simulink model "MotorControl"  (R2023b)
settings: Solver=FixedStepDiscrete  StartTime=0.0  StopTime=8  FixedStep=1e-5  RelTol=1e-3
libraries: slpidlib x2, autolibpmsminterior x1, autolibinverter x1
settings Model: Creator=Elio  LastModifiedBy=Elio

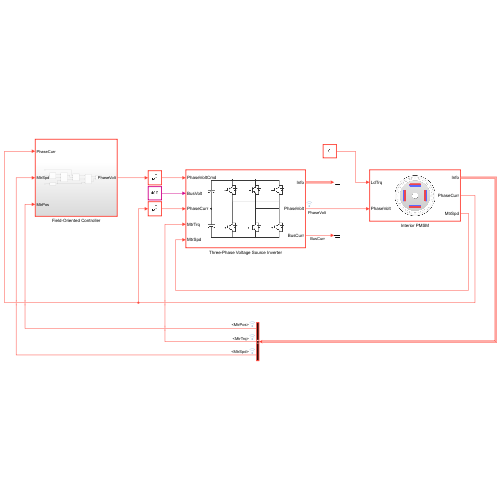
[thumbnail: Simulink's stored preview of the top-level diagram]
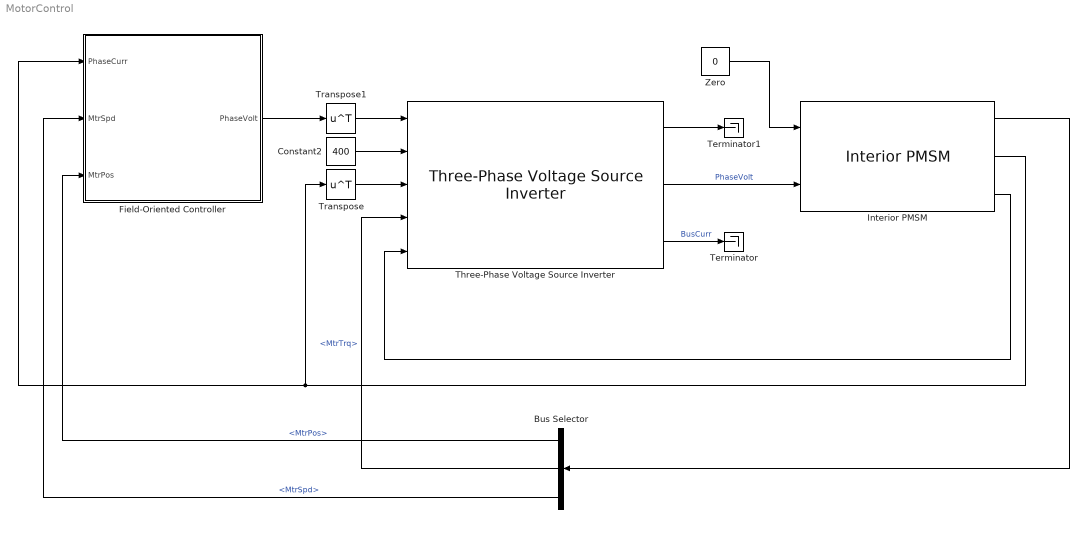
== system MotorControl ==
  Bus Selector : BusSelector  OutputSignals=MtrPos,MtrTrq,MtrSpd
  Constant2 : Constant  Value=400
  Field-Oriented Controller : Subsystem
  Interior PMSM : autolibpmsminterior/Interior PMSM  port_config=Torque  sim_type=Discrete  Ts=1e-5  FilePath=interiorpmsm_motordata.m  P=6  Rs=0.00423  Ldq=[0.171e-3 0.391e-3]  KConstText=Back-emf constant (Ke):  lambda_pm=0.1194  Ke=59.16664  mechanical=[0.0036, 0.0011, 0]  idq0=[0 0]  theta_init=0  omega_init=0  KConst=59.16664  lambda_pm_calc=0.054367  Kt=1.323  RefBlkName='autolibpmsminterior/Interior PMSM'  aMode=1
      settings: LibrarySourceBlock=autolibemachines/Interior PMSM
  Terminator : Terminator
  Terminator1 : Terminator
  Three-Phase Voltage Source Inverter : autolibinverter/Three-Phase Voltage Source Inverter  InvrtrTmpInpEnbl=off  enable_hdl=off  model_type=Commanded phase voltage  fs=10000  w_eff_bp=[-1000 -500 0 500 1000]  n1=128  T_eff_bp=[-200 -100 0 100 200]  Temp_eff_bp=[213.15 293.15 373.15]  n2=128  ploss_table=[1 0.999 0.989 0.997 0.996;0.995 0.994 0.993 0.992 0.991;0.990 0.989 0.988 0.987 0.986;0.985 0.984 0.983 0.982 0.981;0.980 0.979 0.978 0.977 0.976]  ploss_table_3d=cat(3,0.95*[1 0.999 0.989 0.997 0.996;0.995 0.994 0.993 0.992 0.991;0.990 0.989 0.988 0.987 0.986;0.985 0.984 0.983 0.982 0.981;0.980 0.979 0.978 0.977 0.976],[1 0.999 0.989 0.997 0.996;0.995 0.994 0.993 0.992 0.991;0.990 0.989 0.988 0.987 0.986;0.985 0.984 0.983 0.982 0.981;0.980 0.979 0.978 0.977 0.976],0.92*[1 0.999 0.989 0.997 0.996;0.995 0.994 0.993 0.992 0.991;0.990 0.989 0.988 0.987 0.986;0.985 0.984 0.983 0.982 0.981;0.980 0.979 0.978 0.977 0.976])  preExtrapFlag=off  u1max=1000  u1min=-1000  u2max=200  u2min=-200  intPrec=23  RefBlkName='autolibmappedmotor/Mapped Motor'  CalLossMapData={}  CalLossWithTempMapData={}
      settings: LibrarySourceBlock=autolibemachines/Three-Phase Voltage Source Inverter
  Transpose : Math  Operator=transpose
  Transpose1 : Math  Operator=transpose
  Zero : Constant  Value=0  OutDataTypeStr=Inherit: Inherit via back propagation  SampleTime=1e-5
  wires:
  Zero/1 -> Interior PMSM/1
  Interior PMSM/2 -> Transpose/1, Field-Oriented Controller/1(PhaseCurr)
  Three-Phase Voltage Source Inverter/2 -> Interior PMSM/2  "PhaseVolt"
  Bus Selector/1 -> Field-Oriented Controller/3(MtrPos)  "<MtrPos>"
  Three-Phase Voltage Source Inverter/1 -> Terminator1/1
  Bus Selector/3 -> Field-Oriented Controller/2(MtrSpd)  "<MtrSpd>"
  Transpose/1 -> Three-Phase Voltage Source Inverter/3
  Bus Selector/2 -> Three-Phase Voltage Source Inverter/4  "<MtrTrq>"
  Transpose1/1 -> Three-Phase Voltage Source Inverter/1
  Constant2/1 -> Three-Phase Voltage Source Inverter/2
  Three-Phase Voltage Source Inverter/3 -> Terminator/1  "BusCurr"
  Field-Oriented Controller/1(PhaseVolt) -> Transpose1/1
  Interior PMSM/3 -> Three-Phase Voltage Source Inverter/5
  Interior PMSM/1 -> Bus Selector/1

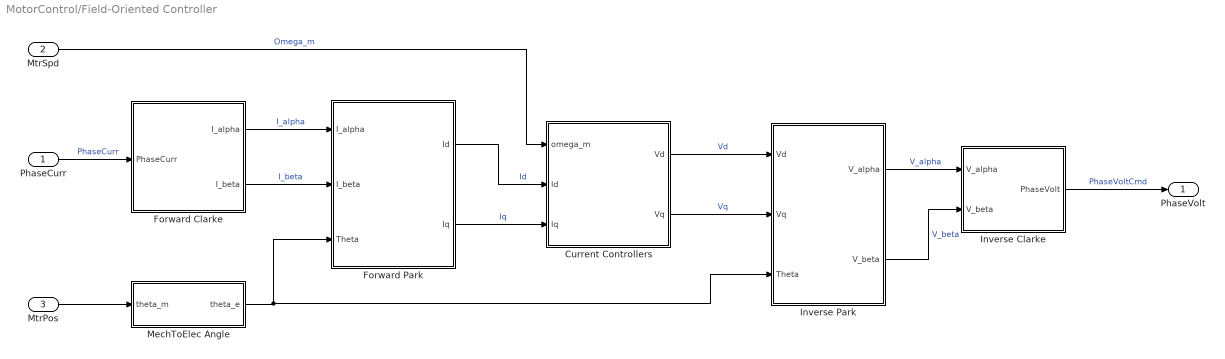
== system MotorControl/Field-Oriented Controller ==
  PhaseCurr : Inport
  MtrSpd : Inport  Port=2
  MtrPos : Inport  Port=3
  Current Controllers : Subsystem
  Forward Clarke : Subsystem
  Forward Park : Subsystem
  Inverse Clarke : Subsystem
  Inverse Park : Subsystem
  MechToElec Angle : Subsystem
  PhaseVolt : Outport
  wires:
  PhaseCurr/1 -> Forward Clarke/1(PhaseCurr)  "PhaseCurr"
  Forward Clarke/1(I_alpha) -> Forward Park/1(I_alpha)  "I_alpha"
  Forward Clarke/2(I_beta) -> Forward Park/2(I_beta)  "I_beta"
  MtrPos/1 -> MechToElec Angle/1(theta_m)
  Inverse Clarke/1(PhaseVolt) -> PhaseVolt/1  "PhaseVoltCmd"
  MtrSpd/1 -> Current Controllers/1(omega_m)  "Omega_m"
  Inverse Park/2(V_beta) -> Inverse Clarke/2(V_beta)  "V_beta"
  Inverse Park/1(V_alpha) -> Inverse Clarke/1(V_alpha)  "V_alpha"
  Forward Park/1(Id) -> Current Controllers/2(Id)  "Id"
  Forward Park/2(Iq) -> Current Controllers/3(Iq)  "Iq"
  Current Controllers/1(Vd) -> Inverse Park/1(Vd)  "Vd"
  Current Controllers/2(Vq) -> Inverse Park/2(Vq)  "Vq"
  MechToElec Angle/1(theta_e) -> Forward Park/3(Theta), Inverse Park/3(Theta)

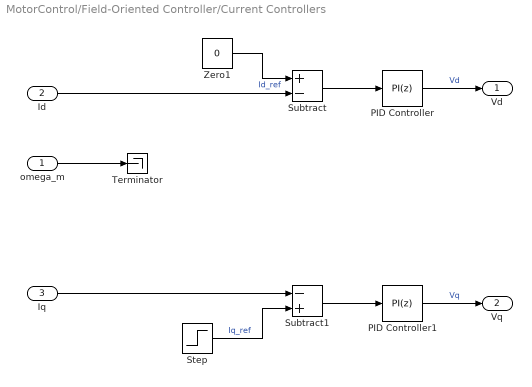
== system MotorControl/Field-Oriented Controller/Current Controllers ==
  omega_m : Inport
  Id : Inport  Port=2
  Iq : Inport  Port=3
  PID Controller : slpidlib/PID Controller  Controller=PI  Form=Parallel  TimeDomain=Discrete-time  UseExternalTs=off  SampleTime=1e-5  IntegratorMethod=Forward Euler  FilterMethod=Forward Euler  ControllerParametersSource=internal  P=13.4666695236978  I=8567.48164264561  UseKiTs=off  D=0  N=100  UseFilter=on  TunerSelectOption=Transfer Function Based (PID Tuner App)  InitialConditionSource=internal  InitialConditionForIntegrator=0  InitialConditionForFilter=0  DifferentiatorICPrevScaledInput=0  ExternalReset=none  TrackingMode=off  Kt=1  LimitOutput=off  SatLimitsSource=internal  UpperSaturationLimit=inf  LowerSaturationLimit=-inf  LinearizeAsGain=on  AntiWindupMode=none  Kb=1  LimitIntegrator=off  UpperIntegratorSaturationLimit=inf  LowerIntegratorSaturationLimit=-inf  POutMin=[]  POutMax=[]  IOutMin=[]  IOutMax=[]  DOutMin=[]  DOutMax=[]  NOutMin=[]  NOutMax=[]  SumOutMin=[]  SumOutMax=[]  SaturationOutMin=[]  SaturationOutMax=[]  PParamMin=[]  PParamMax=[]  IParamMin=[]  IParamMax=[]  DParamMin=[]  DParamMax=[]  NParamMin=[]  NParamMax=[]  KbParamMin=[]  KbParamMax=[]  KtParamMin=[]  KtParamMax=[]  KbOutMin=[]  KbOutMax=[]  KtOutMin=[]  KtOutMax=[]  IntegratorOutMin=[]  IntegratorOutMax=[]  FilterOutMin=[]  FilterOutMax=[]  SumI1OutMin=[]  SumI1OutMax=[]  SumI2OutMin=[]  SumI2OutMax=[]  SumI3OutMin=[]  SumI3OutMax=[]  SumI4OutMin=[]  SumI4OutMax=[]  SumDOutMin=[]  SumDOutMax=[]  DifferentiatorOutMin=[]  DifferentiatorOutMax=[]  FilterDiffOutCoefMin=[]  FilterDiffOutCoefMax=[]  ReciprocalOutMin=[]  ReciprocalOutMax=[]  SumDenOutMin=[]  SumDenOutMax=[]  SumNumOutMin=[]  SumNumOutMax=[]  DivideOutMin=[]  DivideOutMax=[]  UdiffTsProdOutMin=[]  UdiffTsProdOutMax=[]  NTsProdOutMin=[]  NTsProdOutMax=[]  UintegralTsProdOutMin=[]  UintegralTsProdOutMax=[]  UngainTsProdOutMin=[]  UngainTsProdOutMax=[]  ClampingZeroOutDataTypeStr=Inherit: Inherit via back propagation  ClampingZeroOutMin=[]  ClampingZeroOutMax=[]  FilterDenConstantOutDataTypeStr=Inherit: Inherit via back propagation  FilterDenConstantOutMin=[]  FilterDenConstantOutMax=[]  PCopyOutDataTypeStr=Inherit: Inherit via back propagation  PCopyOutMin=[]  PCopyOutMax=[]  NCopyOutDataTypeStr=Inherit: Inherit via back propagation  NCopyOutMin=[]  NCopyOutMax=[]  IntegratorContinuousStateAttributes=''  IntegratorStateMustResolveToSignalObject=off  IntegratorRTWStateStorageClass=Auto  FilterContinuousStateAttributes=''  FilterStateMustResolveToSignalObject=off  FilterRTWStateStorageClass=Auto  ParallelPVariant=InternalParameters  IdealPVariant=Disabled  IVariant=InternalParameters  DVariant=Disabled  IntegratorVariant=Discrete  SatVariant=Disabled  AWVariant=Passthrough  PCopyVariant=Disabled  TRVariant=Disabled  FdbkBlocksVariant=Forward  IdealPFdbkVariant=Disabled  SatFdbkVariant=Disabled  DerivativeFilterVariant=Disabled  NVariant=Disabled  NCopyVariant=Disabled_SignalSpec  FilterICVariant=Disabled  IntegratorICVariant=InternalICs  ExternalResetVariant=Disabled  TRSumVariant=Passthrough  SumFdbkVariant=Disabled  SumVariant=Sum_PI  TsampFilterVariant=InternalTs  TsampNgainVariant=Passthrough  TsampIntegralVariant=Disabled_SignalSpec  ExternalSaturationOutDataTypeStr=Inherit: Same as second input
  PID Controller1 : slpidlib/PID Controller  Controller=PI  Form=Parallel  TimeDomain=Discrete-time  UseExternalTs=off  SampleTime=1e-5  IntegratorMethod=Forward Euler  FilterMethod=Forward Euler  ControllerParametersSource=internal  P=25  I=13000  UseKiTs=off  D=0  N=100  UseFilter=on  TunerSelectOption=Transfer Function Based (PID Tuner App)  InitialConditionSource=internal  InitialConditionForIntegrator=0  InitialConditionForFilter=0  DifferentiatorICPrevScaledInput=0  ExternalReset=none  TrackingMode=off  Kt=1  LimitOutput=off  SatLimitsSource=internal  UpperSaturationLimit=inf  LowerSaturationLimit=-inf  LinearizeAsGain=on  AntiWindupMode=none  Kb=1  LimitIntegrator=off  UpperIntegratorSaturationLimit=inf  LowerIntegratorSaturationLimit=-inf  POutMin=[]  POutMax=[]  IOutMin=[]  IOutMax=[]  DOutMin=[]  DOutMax=[]  NOutMin=[]  NOutMax=[]  SumOutMin=[]  SumOutMax=[]  SaturationOutMin=[]  SaturationOutMax=[]  PParamMin=[]  PParamMax=[]  IParamMin=[]  IParamMax=[]  DParamMin=[]  DParamMax=[]  NParamMin=[]  NParamMax=[]  KbParamMin=[]  KbParamMax=[]  KtParamMin=[]  KtParamMax=[]  KbOutMin=[]  KbOutMax=[]  KtOutMin=[]  KtOutMax=[]  IntegratorOutMin=[]  IntegratorOutMax=[]  FilterOutMin=[]  FilterOutMax=[]  SumI1OutMin=[]  SumI1OutMax=[]  SumI2OutMin=[]  SumI2OutMax=[]  SumI3OutMin=[]  SumI3OutMax=[]  SumI4OutMin=[]  SumI4OutMax=[]  SumDOutMin=[]  SumDOutMax=[]  DifferentiatorOutMin=[]  DifferentiatorOutMax=[]  FilterDiffOutCoefMin=[]  FilterDiffOutCoefMax=[]  ReciprocalOutMin=[]  ReciprocalOutMax=[]  SumDenOutMin=[]  SumDenOutMax=[]  SumNumOutMin=[]  SumNumOutMax=[]  DivideOutMin=[]  DivideOutMax=[]  UdiffTsProdOutMin=[]  UdiffTsProdOutMax=[]  NTsProdOutMin=[]  NTsProdOutMax=[]  UintegralTsProdOutMin=[]  UintegralTsProdOutMax=[]  UngainTsProdOutMin=[]  UngainTsProdOutMax=[]  ClampingZeroOutDataTypeStr=Inherit: Inherit via back propagation  ClampingZeroOutMin=[]  ClampingZeroOutMax=[]  FilterDenConstantOutDataTypeStr=Inherit: Inherit via back propagation  FilterDenConstantOutMin=[]  FilterDenConstantOutMax=[]  PCopyOutDataTypeStr=Inherit: Inherit via back propagation  PCopyOutMin=[]  PCopyOutMax=[]  NCopyOutDataTypeStr=Inherit: Inherit via back propagation  NCopyOutMin=[]  NCopyOutMax=[]  IntegratorContinuousStateAttributes=''  IntegratorStateMustResolveToSignalObject=off  IntegratorRTWStateStorageClass=Auto  FilterContinuousStateAttributes=''  FilterStateMustResolveToSignalObject=off  FilterRTWStateStorageClass=Auto  ParallelPVariant=InternalParameters  IdealPVariant=Disabled  IVariant=InternalParameters  DVariant=Disabled  IntegratorVariant=Discrete  SatVariant=Disabled  AWVariant=Passthrough  PCopyVariant=Disabled  TRVariant=Disabled  FdbkBlocksVariant=Forward  IdealPFdbkVariant=Disabled  SatFdbkVariant=Disabled  DerivativeFilterVariant=Disabled  NVariant=Disabled  NCopyVariant=Disabled_SignalSpec  FilterICVariant=Disabled  IntegratorICVariant=InternalICs  ExternalResetVariant=Disabled  TRSumVariant=Passthrough  SumFdbkVariant=Disabled  SumVariant=Sum_PI  TsampFilterVariant=InternalTs  TsampNgainVariant=Passthrough  TsampIntegralVariant=Disabled_SignalSpec  ExternalSaturationOutDataTypeStr=Inherit: Same as second input
  Step : Step  After=30  SampleTime=1e-5
  Subtract : Sum  Inputs=+-
  Subtract1 : Sum  Inputs=-+
  Terminator : Terminator
  Zero1 : Constant  Value=0  OutDataTypeStr=Inherit: Inherit via back propagation
  Vd : Outport
  Vq : Outport  Port=2
  wires:
  Subtract1/1 -> PID Controller1/1
  Step/1 -> Subtract1/2  "Iq_ref"
  Zero1/1 -> Subtract/1  "Id_ref"
  Subtract/1 -> PID Controller/1
  Id/1 -> Subtract/2
  Iq/1 -> Subtract1/1
  PID Controller/1 -> Vd/1  "Vd"
  PID Controller1/1 -> Vq/1  "Vq"
  omega_m/1 -> Terminator/1

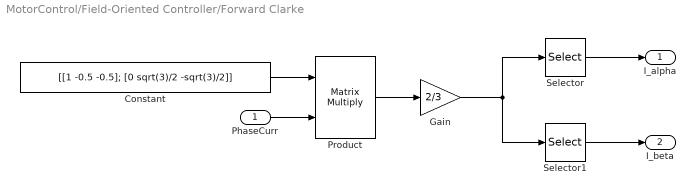
== system MotorControl/Field-Oriented Controller/Forward Clarke ==
  PhaseCurr : Inport
  Constant : Constant  Value=[[1 -0.5 -0.5]; [0 sqrt(3)/2 -sqrt(3)/2]]  SampleTime=1e-5
  Gain : Gain  Gain=2/3
  Product : Product  Multiplication=Matrix(*)
  Selector : Selector  InputPortWidth=2  IndexOptions=Index vector (dialog)  Indices=1  OutputSizes=1
  Selector1 : Selector  InputPortWidth=2  IndexOptions=Index vector (dialog)  Indices=2  OutputSizes=1
  I_alpha : Outport
  I_beta : Outport  Port=2
  wires:
  Constant/1 -> Product/1
  Product/1 -> Gain/1
  Gain/1 -> Selector1/1, Selector/1
  Selector/1 -> I_alpha/1
  Selector1/1 -> I_beta/1
  PhaseCurr/1 -> Product/2

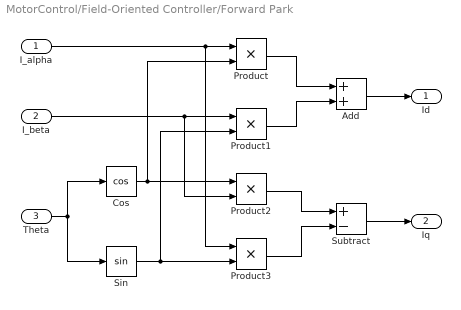
== system MotorControl/Field-Oriented Controller/Forward Park ==
  I_alpha : Inport
  I_beta : Inport  Port=2
  Theta : Inport  Port=3
  Add : Sum
  Cos : Trigonometry  Operator=cos
  Product{,1..3} (4 alike) : Product
  Sin : Trigonometry
  Subtract : Sum  Inputs=+-
  Id : Outport
  Iq : Outport  Port=2
  wires:
  Theta/1 -> Sin/1, Cos/1
  I_alpha/1 -> Product/1, Product3/1
  Cos/1 -> Product2/1, Product/2
  I_beta/1 -> Product1/1, Product2/2
  Sin/1 -> Product3/2, Product1/2
  Product/1 -> Add/1
  Product1/1 -> Add/2
  Add/1 -> Id/1
  Product2/1 -> Subtract/1
  Product3/1 -> Subtract/2
  Subtract/1 -> Iq/1

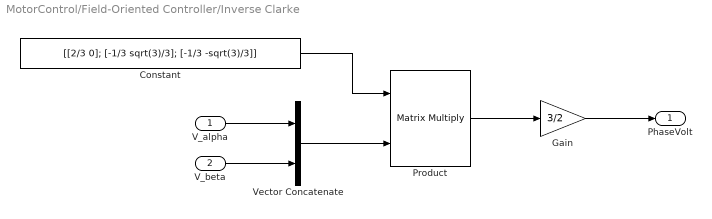
== system MotorControl/Field-Oriented Controller/Inverse Clarke ==
  V_alpha : Inport
  V_beta : Inport  Port=2
  Constant : Constant  Value=[[2/3 0]; [-1/3 sqrt(3)/3]; [-1/3 -sqrt(3)/3]]  SampleTime=1e-5
  Gain : Gain  Gain=3/2
  Product : Product  Multiplication=Matrix(*)
  Vector Concatenate : Concatenate
  PhaseVolt : Outport
  wires:
  V_alpha/1 -> Vector Concatenate/1
  V_beta/1 -> Vector Concatenate/2
  Vector Concatenate/1 -> Product/2
  Constant/1 -> Product/1
  Product/1 -> Gain/1
  Gain/1 -> PhaseVolt/1

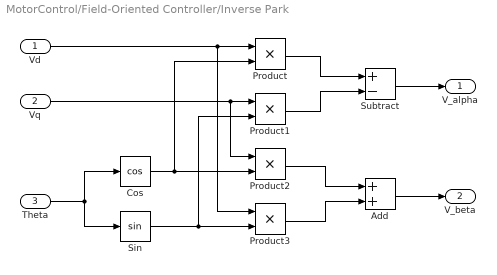
== system MotorControl/Field-Oriented Controller/Inverse Park ==
  Vd : Inport
  Vq : Inport  Port=2
  Theta : Inport  Port=3
  Add : Sum
  Cos : Trigonometry  Operator=cos
  Product{,1..3} (4 alike) : Product
  Sin : Trigonometry
  Subtract : Sum  Inputs=+-
  V_alpha : Outport
  V_beta : Outport  Port=2
  wires:
  Theta/1 -> Cos/1, Sin/1
  Vd/1 -> Product3/1, Product/1
  Cos/1 -> Product/2, Product2/2
  Vq/1 -> Product2/1, Product1/1
  Sin/1 -> Product1/2, Product3/2
  Product/1 -> Subtract/1
  Product1/1 -> Subtract/2
  Subtract/1 -> V_alpha/1
  Product2/1 -> Add/1
  Product3/1 -> Add/2
  Add/1 -> V_beta/1

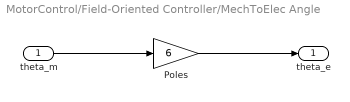
== system MotorControl/Field-Oriented Controller/MechToElec Angle ==
  theta_m : Inport
  Poles : Gain  Gain=6
  theta_e : Outport
  wires:
  theta_m/1 -> Poles/1
  Poles/1 -> theta_e/1
